simulink model "ACC"  (R2023b)
settings: Solver=VariableStepAuto  StartTime=0.0  StopTime=10.0  RelTol=1e-3
undefined symbols (not defined in the file or in its folder): driver_I, driver_P, driving, egoID, lr, m, matlabshared, R, tau, Ts, yawerr_gain
libraries: drivingscenarioandsensors x3, slpidlib x1, autolibshared x1
settings Model: Creator=USER  LastModifiedBy=USER

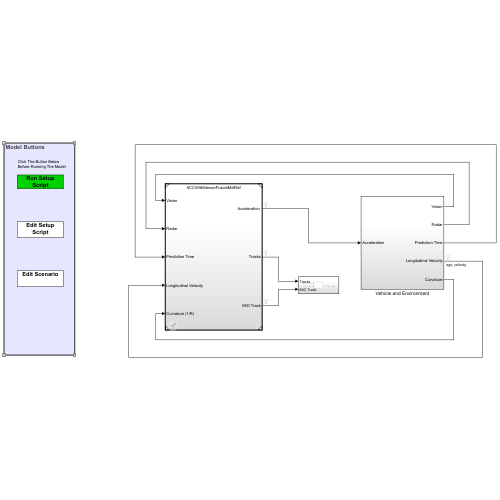
[thumbnail: Simulink's stored preview of the top-level diagram]
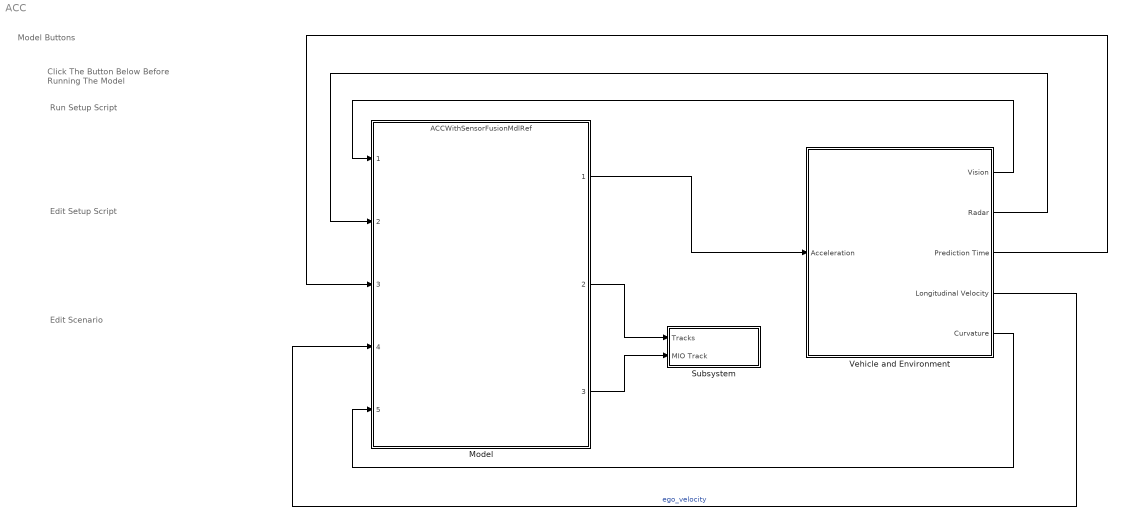
== system ACC ==
  note: Model Buttons
  note: Run Setup Script
  note: Edit Setup Script
  note: Edit Scenario
  note: Click The Button Below Before Running The Model
  Model : ModelReference  ModelNameDialog=ACCWithSensorFusionMdlRef  SimulationMode=Normal  ModelReferenceVersion=7.0
  Subsystem : Subsystem
  Vehicle and Environment : Subsystem
  wires:
  Vehicle and Environment/5(Curvature) -> Model/5
  Vehicle and Environment/1(Vision) -> Model/1
  Model/3 -> Subsystem/2(MIO Track)
  Vehicle and Environment/3(Prediction Time) -> Model/3
  Model/1 -> Vehicle and Environment/1(Acceleration)
  Model/2 -> Subsystem/1(Tracks)
  Vehicle and Environment/2(Radar) -> Model/2
  Vehicle and Environment/4(Longitudinal Velocity) -> Model/4  "ego_velocity"

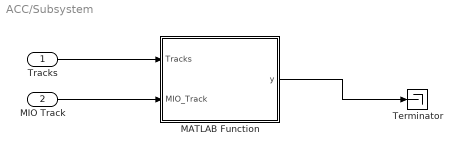
== system ACC/Subsystem ==
  Tracks : Inport
  MIO Track : Inport  Port=2
  MATLAB Function : MATLAB Function  TreatAsAtomicUnit=on
  Terminator : Terminator
  wires:
  MATLAB Function/1(y) -> Terminator/1
  Tracks/1 -> MATLAB Function/1(Tracks)
  MIO Track/1 -> MATLAB Function/2(MIO_Track)

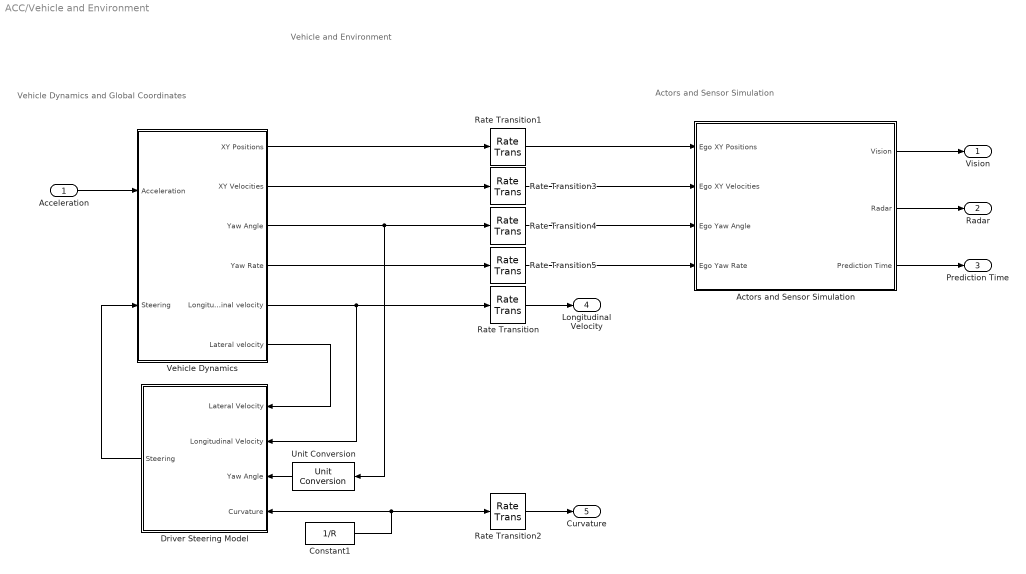
== system ACC/Vehicle and Environment ==
  note: Actors and Sensor Simulation
  note: Vehicle and Environment
  note: Vehicle Dynamics and Global Coordinates
  Acceleration : Inport  OutDataTypeStr=double  PortDimensions=1
  Actors and Sensor Simulation : Subsystem
  Constant1 : Constant  Value=1/R
  Driver Steering Model : Subsystem
  Rate Transition{,1..5} (6 alike) : RateTransition  OutPortSampleTime=Ts
  Unit Conversion : UnitConversion
  Vehicle Dynamics : Subsystem  VariantControl=Variant2
  Vision : Outport  VectorParamsAs1DForOutWhenUnconnected=off
  Radar : Outport  Port=2  VectorParamsAs1DForOutWhenUnconnected=off
  Prediction Time : Outport  Port=3  VectorParamsAs1DForOutWhenUnconnected=off
  Longitudinal Velocity : Outport  Port=4  VectorParamsAs1DForOutWhenUnconnected=off
  Curvature : Outport  Port=5  VectorParamsAs1DForOutWhenUnconnected=off
  wires:
  Actors and Sensor Simulation/1(Vision) -> Vision/1
  Actors and Sensor Simulation/2(Radar) -> Radar/1
  Actors and Sensor Simulation/3(Prediction Time) -> Prediction Time/1
  Rate Transition1/1 -> Actors and Sensor Simulation/1(Ego XY Positions)
  Rate Transition3/1 -> Actors and Sensor Simulation/2(Ego XY Velocities)
  Rate Transition4/1 -> Actors and Sensor Simulation/3(Ego Yaw Angle)
  Rate Transition5/1 -> Actors and Sensor Simulation/4(Ego Yaw Rate)
  Rate Transition2/1 -> Curvature/1
  Unit Conversion/1 -> Driver Steering Model/3(Yaw Angle)
  Vehicle Dynamics/4(Yaw Rate) -> Rate Transition5/1
  Vehicle Dynamics/3(Yaw Angle) -> Rate Transition4/1, Unit Conversion/1
  Vehicle Dynamics/6(Lateral velocity) -> Driver Steering Model/1(Lateral Velocity)
  Vehicle Dynamics/5(Longitudinal velocity) -> Rate Transition/1, Driver Steering Model/2(Longitudinal Velocity)
  Rate Transition/1 -> Longitudinal Velocity/1
  Driver Steering Model/1(Steering) -> Vehicle Dynamics/2(Steering)
  Acceleration/1 -> Vehicle Dynamics/1(Acceleration)
  Constant1/1 -> Driver Steering Model/4(Curvature), Rate Transition2/1
  Vehicle Dynamics/1(XY Positions) -> Rate Transition1/1
  Vehicle Dynamics/2(XY Velocities) -> Rate Transition3/1

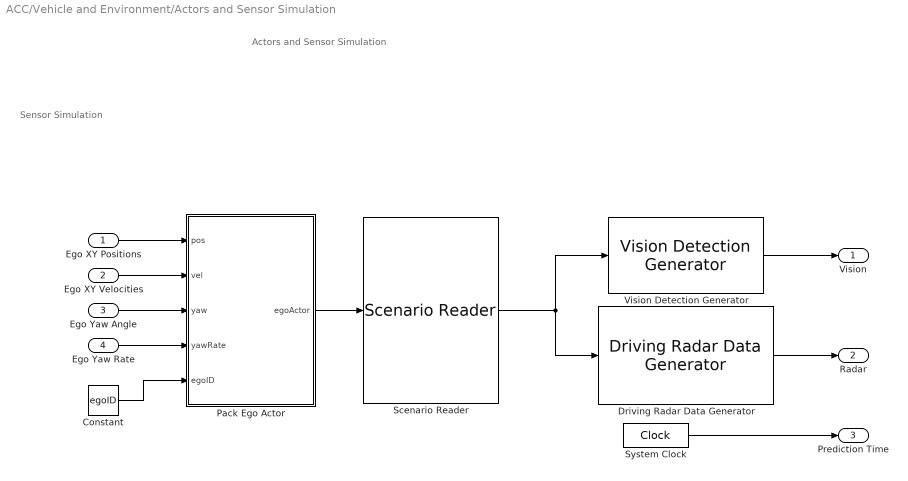
== system ACC/Vehicle and Environment/Actors and Sensor Simulation ==
  note: Sensor Simulation
  note: Actors and Sensor Simulation
  Ego XY Positions : Inport
  Ego XY Velocities : Inport  Port=2
  Ego Yaw Angle : Inport  Port=3
  Ego Yaw Rate : Inport  Port=4
  Constant : Constant  Value=egoID
  Driving Radar Data Generator : drivingscenarioandsensors/Driving Radar Data Generator  SensorIndex=2  UpdateRate=10  MountingLocation=[ 3.7, 0, 0.2 ]  MountingAngles=[0 0 0]  HasElevation=off  HasRangeRate=on  HasNoise=on  HasFalseAlarms=on  HasOcclusion=on  MaxNumReportsSource=Property  MaxNumReports=50  TargetReportFormat=Clustered detections  DetectionCoordinates=Body  TrackCoordinates=Body  BusNameSource=Property  BusName=BusRadar  AzimuthResolution=4  ElevationResolution=5  RangeResolution=2.5  RangeRateResolution=0.5  AzimuthBiasFraction=0.1  ElevationBiasFraction=0.1  RangeBiasFraction=0.05  RangeRateBiasFraction=0.05  FieldOfView=[ 20, 5 ]  RangeLimits=[ 0, 174 ]  RangeRateLimits=[ -100, 100 ]  DetectionProbability=0.9  FalseAlarmRate=1e-06  ReferenceRange=100  ReferenceRCS=0  CenterFrequency=77e9  FilterInitializationFcn=initcvekf  ConfirmationThreshold=[2 3]  DeletionThreshold=[5 5]  InitialSeedSource=Repeatable  InitialSeed=0  UsedSeed=matlabshared.tracking.internal.SimulinkUtilities.seedManager(gcb)  ProfilesSource=Parameters  ProfilesParameters=driving.internal.ActorProfilesRadarParameters  ProfilesExpression=struct('ClassID',0,'Length',4.7,'Width',1.8,'Height',1.4,'OriginOffset',[-1.35 0 0],'RCSPattern',[10 10;10 10],'RCSAzimuthAngles',[-180 180],'RCSElevationAngles',[-90 90])
  Pack Ego Actor : MATLAB Function  TreatAsAtomicUnit=on
  Scenario Reader : drivingscenarioandsensors/Scenario Reader  ScenarioSource=From workspace  ScenarioFileName=ACCTestBenchScenario.mat  ScenarioVariableName=scenario  OutputCoordinateSystem=Vehicle coordinates  EgoVehicleSource=Input port  EgoVehicleActorID=egoID  OrientVehiclesOnRoad=off  OutputEgoVehiclePose=off  OutputEgoVehicleState=off  SampleTime=0.1  LaneBoundaryOutput=None  LaneBoundaryDistance=0:0.5:9.5  LaneBoundaryLocation=Center of lane markings  BusNameSource=Property  BusName=BusActors  BusNumActorsSource=Scenario  BusNumActors=100  BusName2Source=Auto  BusName2=BusLaneBoundaries  BusNumLaneBoundariesSource=Scenario  BusNumLaneBoundaries=10  BusName3Source=Auto  BusName3=BusEgoActor  BusName4Source=Auto  BusName4=BusEgoState  ShowCoordinateLabels=on  SimulateUsing=Interpreted execution
  System Clock : DigitalClock  SampleTime=Ts
  Vision Detection Generator : drivingscenarioandsensors/Vision Detection Generator  SensorIndex=1  DetectorOutput=Objects only  UpdateInterval=0.1  LaneUpdateInterval=0.1  SensorLocation=[ 2.1, 0 ]  Height=1.1  Yaw=0  Pitch=1  Roll=0  BusNameSource=Property  BusName=BusVision  BusName2Source=Auto  BusName2=BusLaneDetections  MaxNumDetectionsSource=Property  MaxNumDetections=20  MaxNumLanesSource=Property  MaxNumLanes=30  DetectionCoordinates=Ego Cartesian  SimulateUsing=Interpreted execution  MaxRange=150  BoundingBoxAccuracy=5  ProcessNoiseIntensity=5  MaxSpeed=50  MaxAllowedOcclusion=0.5  MinObjectImageSize=[ 15, 15 ]  DetectionProbability=0.9  FalsePositivesPerImage=0.1  MinLaneImageSize=[ 20, 5 ]  LaneBoundaryAccuracy=3  HasNoise=on  InitialSeedSource=Repeatable  InitialSeed=0  UsedSeed=driving.internal.SimulinkUtilities.seedManager(gcb)  ActorProfilesSource=Parameters  ActorProfilesParameters=driving.internal.ActorProfilesParameters  ActorProfilesExpression=struct( 'ClassID', 0, 'Length', 4.7, 'Width', 1.8, 'Height', 1.4, 'OriginOffset', [ -1.35, 0, 0 ] )  Intrinsics=driving.internal.cameraIntrinsics
  Vision : Outport  VectorParamsAs1DForOutWhenUnconnected=off
  Radar : Outport  Port=2  VectorParamsAs1DForOutWhenUnconnected=off
  Prediction Time : Outport  Port=3  VectorParamsAs1DForOutWhenUnconnected=off
  wires:
  Scenario Reader/1 -> Driving Radar Data Generator/1, Vision Detection Generator/1
  Vision Detection Generator/1 -> Vision/1
  System Clock/1 -> Prediction Time/1
  Pack Ego Actor/1(egoActor) -> Scenario Reader/1
  Ego XY Positions/1 -> Pack Ego Actor/1(pos)
  Ego XY Velocities/1 -> Pack Ego Actor/2(vel)
  Ego Yaw Angle/1 -> Pack Ego Actor/3(yaw)
  Ego Yaw Rate/1 -> Pack Ego Actor/4(yawRate)
  Driving Radar Data Generator/1 -> Radar/1
  Constant/1 -> Pack Ego Actor/5(egoID)

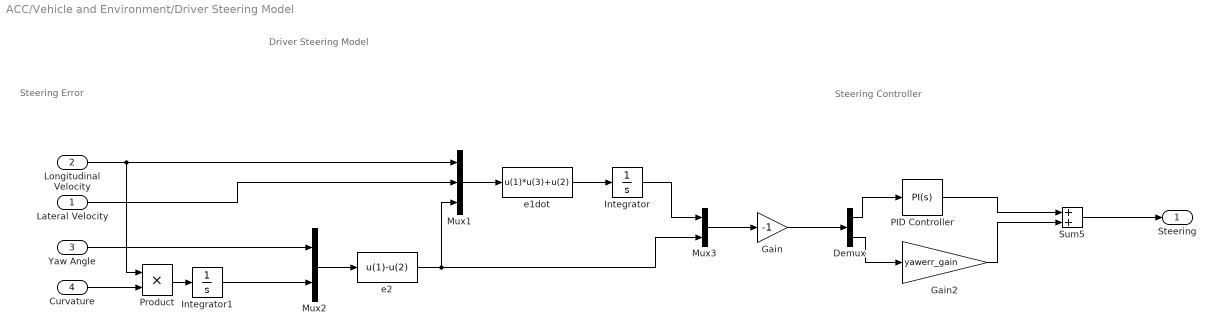
== system ACC/Vehicle and Environment/Driver Steering Model ==
  note: Steering Controller
  note: Steering Error
  note: Driver Steering Model
  Lateral Velocity : Inport
  Longitudinal Velocity : Inport  Port=2
  Yaw Angle : Inport  Port=3  Unit=rad
  Curvature : Inport  Port=4
  Demux : Demux  Outputs=2
  Gain : Gain  Gain=-1
  Gain2 : Gain  Gain=yawerr_gain
  Integrator : Integrator
  Integrator1 : Integrator
  Mux1 : Mux  Inputs=3
  Mux2 : Mux  Inputs=2
  Mux3 : Mux  Inputs=2
  PID Controller : slpidlib/PID Controller  Controller=PI  Form=Parallel  TimeDomain=Continuous-time  UseExternalTs=off  SampleTime=-1  IntegratorMethod=Forward Euler  FilterMethod=Forward Euler  ControllerParametersSource=internal  P=driver_P  I=driver_I  UseKiTs=off  D=0  N=100  UseFilter=on  TunerSelectOption=Transfer Function Based (PID Tuner App)  InitialConditionSource=internal  InitialConditionForIntegrator=0  InitialConditionForFilter=0  DifferentiatorICPrevScaledInput=0  ExternalReset=none  TrackingMode=off  Kt=1  LimitOutput=off  SatLimitsSource=internal  UpperSaturationLimit=inf  LowerSaturationLimit=-inf  LinearizeAsGain=on  AntiWindupMode=none  Kb=1  LimitIntegrator=off  UpperIntegratorSaturationLimit=inf  LowerIntegratorSaturationLimit=-inf  POutMin=[]  POutMax=[]  IOutMin=[]  IOutMax=[]  DOutMin=[]  DOutMax=[]  NOutMin=[]  NOutMax=[]  SumOutMin=[]  SumOutMax=[]  SaturationOutMin=[]  SaturationOutMax=[]  PParamMin=[]  PParamMax=[]  IParamMin=[]  IParamMax=[]  DParamMin=[]  DParamMax=[]  NParamMin=[]  NParamMax=[]  KbParamMin=[]  KbParamMax=[]  KtParamMin=[]  KtParamMax=[]  KbOutMin=[]  KbOutMax=[]  KtOutMin=[]  KtOutMax=[]  IntegratorOutMin=[]  IntegratorOutMax=[]  FilterOutMin=[]  FilterOutMax=[]  SumI1OutMin=[]  SumI1OutMax=[]  SumI2OutMin=[]  SumI2OutMax=[]  SumI3OutMin=[]  SumI3OutMax=[]  SumI4OutMin=[]  SumI4OutMax=[]  SumDOutMin=[]  SumDOutMax=[]  DifferentiatorOutMin=[]  DifferentiatorOutMax=[]  FilterDiffOutCoefMin=[]  FilterDiffOutCoefMax=[]  ReciprocalOutMin=[]  ReciprocalOutMax=[]  SumDenOutMin=[]  SumDenOutMax=[]  SumNumOutMin=[]  SumNumOutMax=[]  DivideOutMin=[]  DivideOutMax=[]  UdiffTsProdOutMin=[]  UdiffTsProdOutMax=[]  NTsProdOutMin=[]  NTsProdOutMax=[]  UintegralTsProdOutMin=[]  UintegralTsProdOutMax=[]  UngainTsProdOutMin=[]  UngainTsProdOutMax=[]  ClampingZeroOutDataTypeStr=Inherit: Inherit via back propagation  ClampingZeroOutMin=[]  ClampingZeroOutMax=[]  FilterDenConstantOutDataTypeStr=Inherit: Inherit via back propagation  FilterDenConstantOutMin=[]  FilterDenConstantOutMax=[]  PCopyOutDataTypeStr=Inherit: Inherit via back propagation  PCopyOutMin=[]  PCopyOutMax=[]  NCopyOutDataTypeStr=Inherit: Inherit via back propagation  NCopyOutMin=[]  NCopyOutMax=[]  IntegratorContinuousStateAttributes=''  IntegratorStateMustResolveToSignalObject=off  IntegratorRTWStateStorageClass=Auto  FilterContinuousStateAttributes=''  FilterStateMustResolveToSignalObject=off  FilterRTWStateStorageClass=Auto  ParallelPVariant=InternalParameters  IdealPVariant=Disabled  IVariant=InternalParameters  DVariant=Disabled  IntegratorVariant=Continuous  SatVariant=Disabled  AWVariant=Passthrough  PCopyVariant=Disabled  TRVariant=Disabled  FdbkBlocksVariant=Forward  IdealPFdbkVariant=Disabled  SatFdbkVariant=Disabled  DerivativeFilterVariant=Disabled  NVariant=Disabled  NCopyVariant=Disabled_SignalSpec  FilterICVariant=Disabled  IntegratorICVariant=InternalICs  ExternalResetVariant=Disabled  TRSumVariant=Passthrough  SumFdbkVariant=Disabled  SumVariant=Sum_PI  TsampFilterVariant=InternalTs  TsampNgainVariant=Passthrough  TsampIntegralVariant=Disabled_SignalSpec  ExternalSaturationOutDataTypeStr=Inherit: Same as second input
  Product : Product
  Sum5 : Sum
  e1dot : Fcn  Expr=u(1)*u(3)+u(2)
  e2 : Fcn  Expr=u(1)-u(2)
  Steering : Outport  VectorParamsAs1DForOutWhenUnconnected=off
  wires:
  e1dot/1 -> Integrator/1
  Mux2/1 -> e2/1
  e2/1 -> Mux1/3, Mux3/2
  Mux3/1 -> Gain/1
  Lateral Velocity/1 -> Mux1/2
  Yaw Angle/1 -> Mux2/1
  Mux1/1 -> e1dot/1
  Integrator/1 -> Mux3/1
  Product/1 -> Integrator1/1
  Integrator1/1 -> Mux2/2
  Curvature/1 -> Product/2
  Longitudinal Velocity/1 -> Product/1, Mux1/1
  Gain2/1 -> Sum5/2
  PID Controller/1 -> Sum5/1
  Demux/2 -> Gain2/1
  Sum5/1 -> Steering/1
  Demux/1 -> PID Controller/1
  Gain/1 -> Demux/1

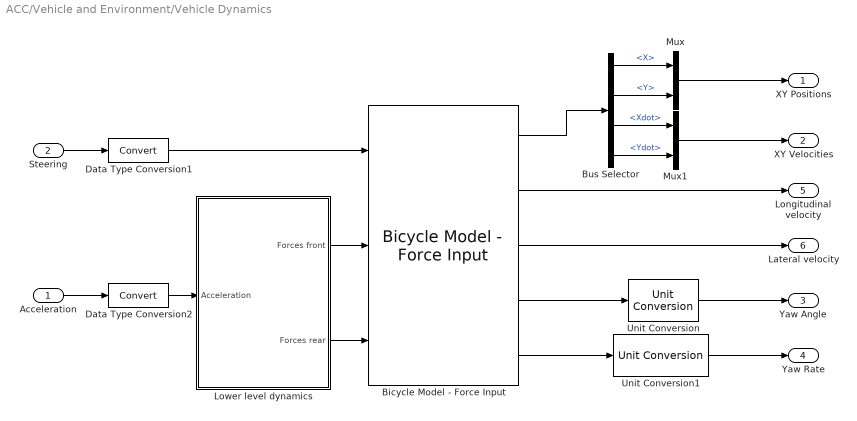
== system ACC/Vehicle and Environment/Vehicle Dynamics ==
  Acceleration : Inport  Unit=m/s^2
  Steering : Inport  Port=2  Unit=rad
  Bicycle Model - Force Input : autolibshared/Bicycle Model - Force Input  trackMode=Single (bicycle)  inputMode=External longitudinal forces  frontSteerMode=on  rearSteerMode=off  windMode=off  muMode=off  extFMode=off  extMMode=off  aMode=3  NF=2  NR=2  m=m  a=lf  b=lr  h=0.35  X_o=x0_ego  xdot_o=v0_ego  CalphaMode=off  sigmaMode=on  w=[1.4,1.4]  Cy_f=Cf  Cy_r=Cr  sigma_f=.1  sigma_r=.1  alpha_f_brk=[-.1 .1]  Cy_f_data=[-9e3 9e3]  alpha_r_brk=[-.1 .1]  Cy_r_data=[-9e3 9e3]  Y_o=y0_ego  ydot_o=0  Izz=Iz  psi_o=0  r_o=0  Af=0  Cd=.3  Cl=.1  Cpm=.1  beta_w=[0:0.01:0.3]  Cs=[0:0.03:0.9]  Cym=[0:0.01:0.3]  Pabs=101325  Tair=273  g=9.81  mu=1  xdot_tol=.01  Fznom=5000  Fxtire_sat=1e6  Fytire_sat=1e6  longOff=0  latOff=0  vertOff=0
      settings: LibrarySourceBlock=drivingscenarioandsensors/Bicycle Model - Force Input
  Bus Selector : BusSelector  OutputSignals=InertFrm.FrntAxl.Disp.X,InertFrm.FrntAxl.Disp.Y,InertFrm.FrntAxl.Vel.Xdot,InertFrm.FrntAxl.Vel.Ydot
  Data Type Conversion1 : DataTypeConversion  SaturateOnIntegerOverflow=off  RndMeth=Floor
  Data Type Conversion2 : DataTypeConversion  SaturateOnIntegerOverflow=off  RndMeth=Floor
  Lower level dynamics : Subsystem
  Mux : Mux  Inputs=2
  Mux1 : Mux  Inputs=2
  Unit Conversion : UnitConversion
  Unit Conversion1 : UnitConversion
  XY Positions : Outport  Unit=m  VectorParamsAs1DForOutWhenUnconnected=off
  XY Velocities : Outport  Port=2  Unit=m/s  VectorParamsAs1DForOutWhenUnconnected=off
  Yaw Angle : Outport  Port=3  Unit=deg  VectorParamsAs1DForOutWhenUnconnected=off
  Yaw Rate : Outport  Port=4  Unit=degree/s  VectorParamsAs1DForOutWhenUnconnected=off
  Longitudinal velocity : Outport  Port=5  VectorParamsAs1DForOutWhenUnconnected=off
  Lateral velocity : Outport  Port=6  VectorParamsAs1DForOutWhenUnconnected=off
  wires:
  Lower level dynamics/2(Forces rear) -> Bicycle Model - Force Input/3
  Lower level dynamics/1(Forces front) -> Bicycle Model - Force Input/2
  Data Type Conversion2/1 -> Lower level dynamics/1(Acceleration)
  Acceleration/1 -> Data Type Conversion2/1
  Steering/1 -> Data Type Conversion1/1
  Bus Selector/1 -> Mux/1  "<X>"
  Bicycle Model - Force Input/4 -> Unit Conversion/1
  Bus Selector/4 -> Mux1/2  "<Ydot>"
  Bus Selector/2 -> Mux/2  "<Y>"
  Bicycle Model - Force Input/2 -> Longitudinal velocity/1
  Bus Selector/3 -> Mux1/1  "<Xdot>"
  Bicycle Model - Force Input/1 -> Bus Selector/1
  Bicycle Model - Force Input/3 -> Lateral velocity/1
  Mux/1 -> XY Positions/1
  Mux1/1 -> XY Velocities/1
  Bicycle Model - Force Input/5 -> Unit Conversion1/1
  Data Type Conversion1/1 -> Bicycle Model - Force Input/1
  Unit Conversion/1 -> Yaw Angle/1
  Unit Conversion1/1 -> Yaw Rate/1

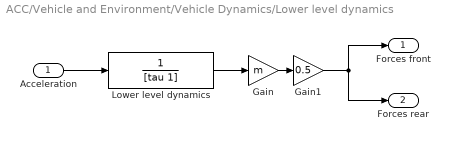
== system ACC/Vehicle and Environment/Vehicle Dynamics/Lower level dynamics ==
  Acceleration : Inport
  Gain : Gain  Gain=m
  Gain1 : Gain  Gain=0.5
  Lower level dynamics : TransferFcn  Denominator=[tau 1]
  Forces front : Outport  VectorParamsAs1DForOutWhenUnconnected=off
  Forces rear : Outport  Port=2  VectorParamsAs1DForOutWhenUnconnected=off
  wires:
  Gain/1 -> Gain1/1
  Gain1/1 -> Forces front/1, Forces rear/1
  Acceleration/1 -> Lower level dynamics/1
  Lower level dynamics/1 -> Gain/1

== matlab function ACC/Subsystem/MATLAB Function ==
  data: Tracks input; y output; MIO_Track input
function y = fcn(Tracks, MIO_Track)
% Extract MIO track and package for visualization in Birds Eye Scope
y = Tracks;
if MIO_Track > 0
    % First track represents MIO
   y.NumTracks = 1;
   Y.Tracks(1) = tracks.Tracks(MIO_Track);
else
    % No valid MIO track
  MIO_Track.NumTracks = 0;
end

== matlab function ACC/Vehicle and Environment/Actors and Sensor Simulation/Pack Ego Actor ==
  data: pos input; egoActor output Bus: BusActorsActors size=1; vel input; yaw input; yawRate input; egoID input
function egoActor = packEgo(pos,vel,yaw,yawRate,egoID)
% Pack ego information into a single ego actor bus


egoActor = struct(...
    'ActorID',egoID,...
    'Position', [pos(1) pos(2) 0], ...
    'Velocity', [vel(1) vel(2) 0], ...
    'Roll', 0, ...
    'Pitch', 0, ...
    'Yaw', yaw, ...
    'AngularVelocity', [0 0 yawRate]);
